simulink model "Simulateur_V8_eq06"  (R2024a)
settings: Solver=FixedStepAuto  StartTime=0.0  StopTime=1  FixedStep=1e-5  RelTol=1e-3
model workspace: external: MATLAB File Simulateur_V7_eq065_saveas.m (data not in the file)
values from neighbouring files (symbols this model uses):
  b = 72.82e-3    (= 0.07282)    [Init.m]    (also in Init_Complet.m)
  E = 18.6e9    (= 18600000000)    [Init.m]    (also in Init_Complet.m)
  h = 1.46e-3    (= 0.00146)    [Init.m]    (also in Init_Complet.m)
  L = 25e-2    (= 0.25)    [Init.m]    (also in Init_Complet.m)
  q = 0.14    [Init.m]    (also in Init_Complet.m)
undefined symbols (not defined in the file or in its folder): c, dens, m
libraries: simulink x3, slpidlib x2
settings Model: SimulationMode=accelerator  Creator=jeann  LastModifiedBy=dadah5
settings RTWCC: GPUComputeCapability=3.5

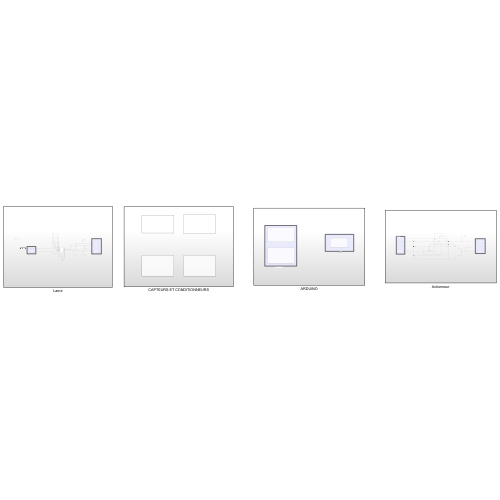
[thumbnail: Simulink's stored preview of the top-level diagram]
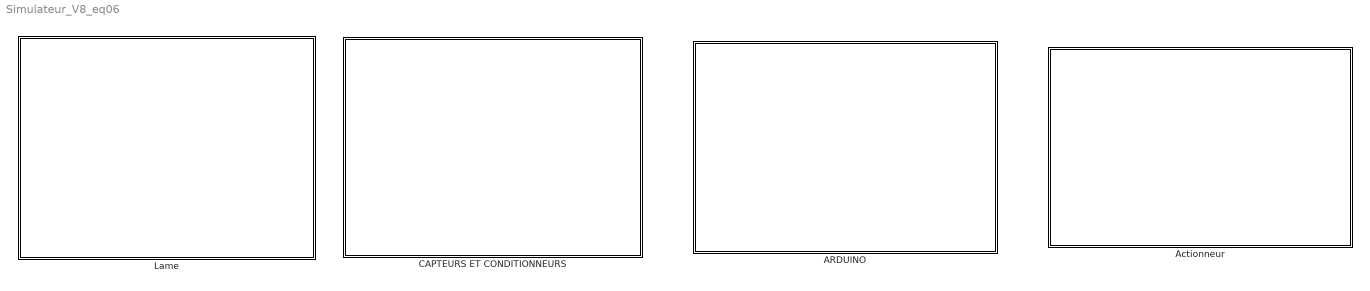
== system Simulateur_V8_eq06 ==
  ARDUINO : Subsystem
  Actionneur : Subsystem
  CAPTEURS ET CONDITIONNEURS : Subsystem
  Lame : Subsystem

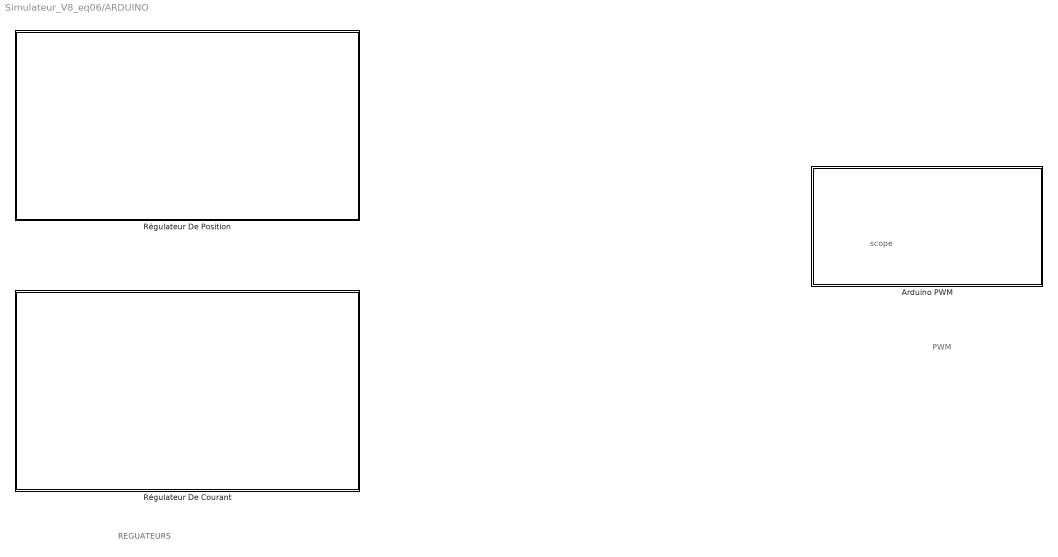
== system Simulateur_V8_eq06/ARDUINO ==
  note: scope
  note: REGUATEURS
  note: PWM
  Arduino PWM : Subsystem
  Régulateur De Courant : Subsystem
  Régulateur De Position : Subsystem

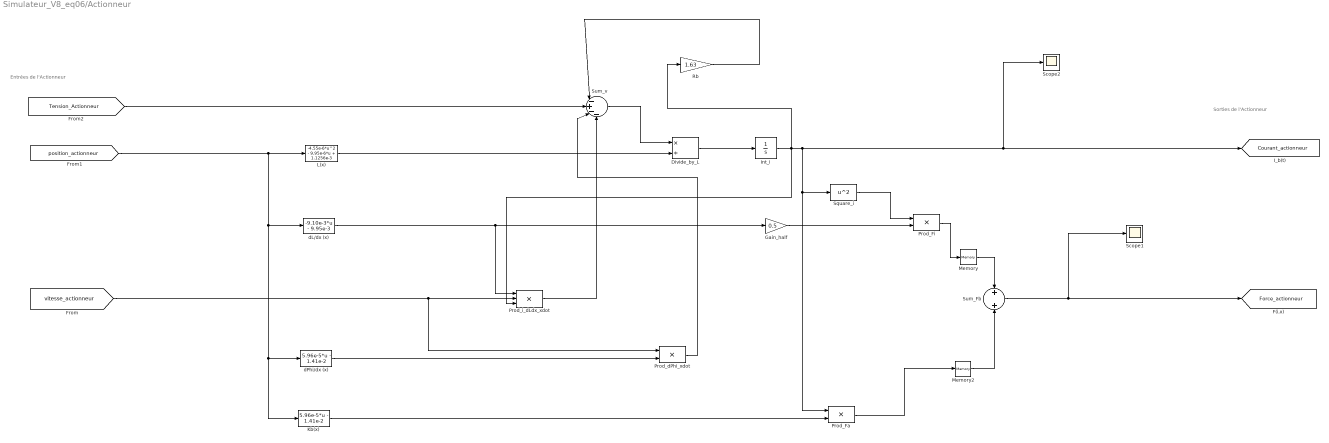
== system Simulateur_V8_eq06/Actionneur ==
  note: Sorties de l'Actionneur
  note: Entrées de l'Actionneur
  Divide_by_L : Product  Inputs=*/
  Gain_half : Gain  Gain=0.5
  Int_i : Integrator
  Kb(x) : Fcn  Expr=5.96e-5*u - 1.41e-2
  L(x) : Fcn  Expr=-4.55e-6*u^2 - 9.95e-6*u + 1.1256e-3
  Memory : Memory
  Memory2 : Memory
  Prod_Fa : Product
  Prod_Fi : Product
  Prod_dPhi_xdot : Product
  Prod_i_dLdx_xdot : Product  Inputs=3
  Rb : Gain  Gain=1.63
  Scope1 : Scope
  Scope2 : Scope
  Square_i : Math  Operator=square
  Sum_Fb : Sum
  Sum_v : Sum  Inputs=|-+--
  dL/dx (x) : Fcn  Expr=-9.10e-3*u - 9.95e-3
  dPhi/dx (x) : Fcn  Expr=5.96e-5*u - 1.41e-2
  tag scope: Courant_actionneur=global, Force_actionneur=global
  wires:
  dL/dx (x)/1 -> Gain_half/1, Prod_i_dLdx_xdot/1
  Sum_Fb/1 -> Scope1/1, [Force_actionneur]
  Rb/1 -> Sum_v/1
  Prod_i_dLdx_xdot/1 -> Sum_v/4
  L(x)/1 -> Divide_by_L/2
  Square_i/1 -> Prod_Fi/1
  Prod_dPhi_xdot/1 -> Sum_v/3
  Gain_half/1 -> Prod_Fi/2
  dPhi/dx (x)/1 -> Prod_dPhi_xdot/2
  Divide_by_L/1 -> Int_i/1
  Int_i/1 -> Prod_i_dLdx_xdot/3, Scope2/1, [Courant_actionneur], Square_i/1, Prod_Fa/1, Rb/1
  Sum_v/1 -> Divide_by_L/1
  [vitesse_actionneur] -> Prod_dPhi_xdot/1, Prod_i_dLdx_xdot/2
  Kb(x)/1 -> Prod_Fa/2
  [position_actionneur] -> dL/dx (x)/1, Kb(x)/1, dPhi/dx (x)/1, L(x)/1
  [Tension_Actionneur] -> Sum_v/2
  Prod_Fi/1 -> Memory/1
  Memory/1 -> Sum_Fb/1
  Prod_Fa/1 -> Memory2/1
  Memory2/1 -> Sum_Fb/2

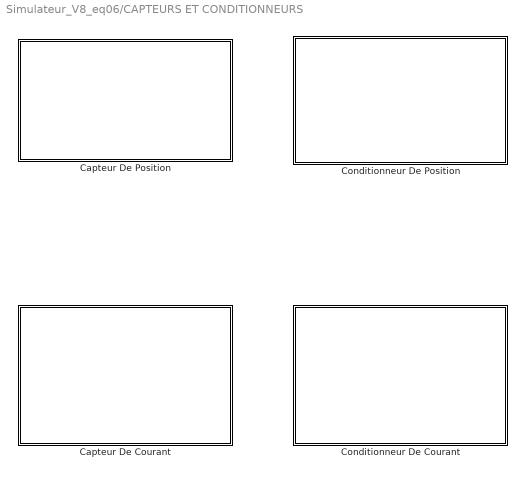
== system Simulateur_V8_eq06/CAPTEURS ET CONDITIONNEURS ==
  Capteur De Courant : Subsystem
  "Capteur De Position " : Subsystem
  Conditionneur De Courant : Subsystem
  Conditionneur De Position : Subsystem

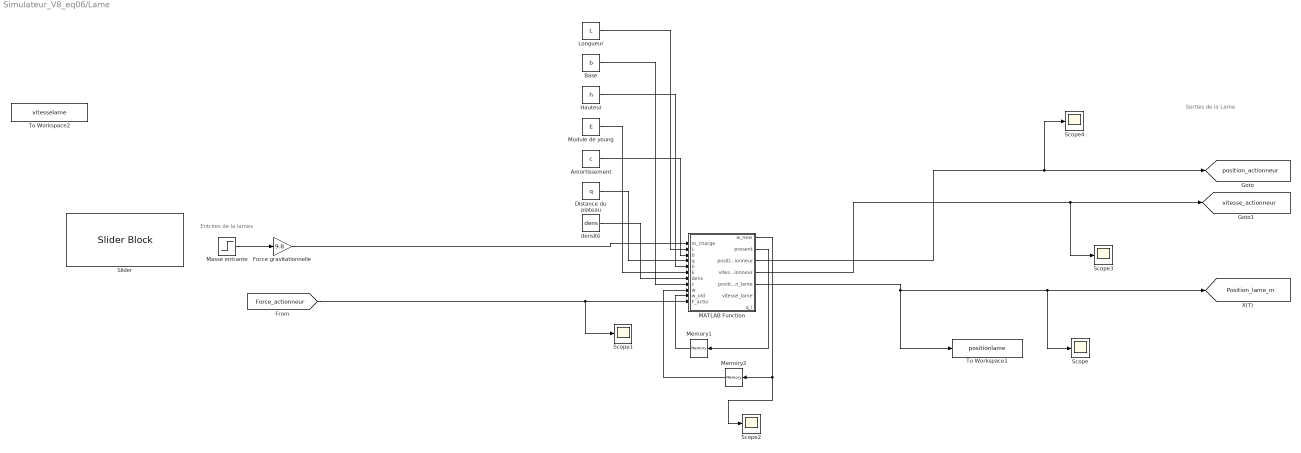
== system Simulateur_V8_eq06/Lame ==
  note: Sorties de la Lame
  note: Entrées de la lames
  Amortissement : Constant  Value=c
  Base : Constant  Value=b
  Distance du plateau : Constant  Value=q
  Force gravitationnelle : Gain  Gain=9.8
  Hauteur : Constant  Value=h
  Longueur : Constant  Value=L
  MATLAB Function : MATLAB Function  TreatAsAtomicUnit=on
  Masse entrante : Step  After=m  SampleTime=3
  Memory1 : Memory  InitialCondition=zeros(12,1)
  Memory2 : Memory  InitialCondition=zeros(12,1)  StateName=matrix
  Module de young : Constant  Value=E
  Scope{,1..4} (5 alike) : Scope
  Slider : SliderBlock
  To Workspace1 : ToWorkspace  VariableName=positionlame  SaveFormat=Timeseries  SampleTime=-1
  To Workspace2 : ToWorkspace  VariableName=vitesselame  SaveFormat=Timeseries  SampleTime=-1
  densité : Constant  Value=dens
  tag scope: Position_lame_m=global, position_actionneur=global, vitesse_actionneur=global
  wires:
  [Force_actionneur] -> Scope1/1, MATLAB Function/11(F_actio)
  MATLAB Function/1(w_new) -> Memory2/1, Scope2/1
  Memory2/1 -> MATLAB Function/9(w)
  MATLAB Function/2(present) -> Memory1/1
  Memory1/1 -> MATLAB Function/10(w_old)
  Hauteur/1 -> MATLAB Function/5(h)
  Module de young/1 -> MATLAB Function/6(E)
  Amortissement/1 -> MATLAB Function/3(b)
  Distance du plateau/1 -> MATLAB Function/4(q)
  densité/1 -> MATLAB Function/7(dens)
  Masse entrante/1 -> Force gravitationnelle/1
  Force gravitationnelle/1 -> MATLAB Function/1(m_charge)
  MATLAB Function/5(position_lame) -> To Workspace1/1, Scope/1, [Position_lame_m]
  MATLAB Function/4(vitesse_actionneur) -> Scope3/1, [vitesse_actionneur]
  MATLAB Function/3(position_actionneur) -> Scope4/1, [position_actionneur]
  Longueur/1 -> MATLAB Function/2(L)
  Base/1 -> MATLAB Function/8(c)

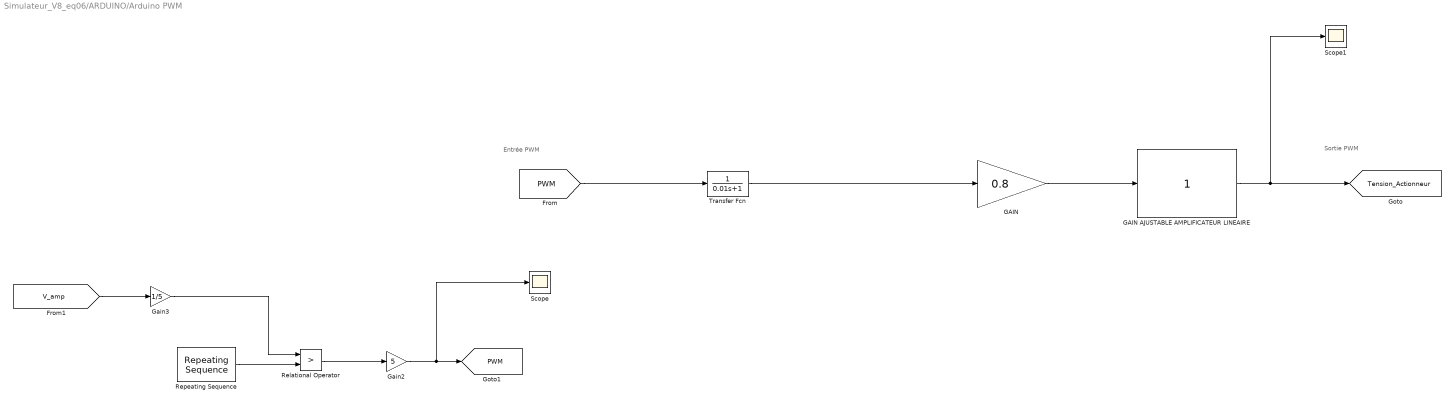
== system Simulateur_V8_eq06/ARDUINO/Arduino PWM ==
  note: Entrée PWM
  note: Sortie PWM
  GAIN : Gain  Gain=0.8
  GAIN AJUSTABLE AMPLIFICATEUR LINEAIRE : simulink/Math Operations/Slider Gain  gain=1  low=1  high=5
  Gain2 : Gain  Gain=5  ParamDataTypeStr=double
  Gain3 : Gain  Gain=1/5
  Relational Operator : RelationalOperator  Operator=>  OutDataTypeStr=boolean  RndMeth=Simplest  InputSameDT=off
  Repeating Sequence : simulink/Sources/Repeating Sequence  rep_seq_t=[0 0.001 0.002]  rep_seq_y=[0 1 0]
  Scope : Scope
  Scope1 : Scope
  Transfer Fcn : TransferFcn  Denominator=[0.01 1]
  tag scope: PWM=global, Tension_Actionneur=global
  wires:
  Transfer Fcn/1 -> GAIN/1
  GAIN AJUSTABLE AMPLIFICATEUR LINEAIRE/1 -> Scope1/1, [Tension_Actionneur]
  GAIN/1 -> GAIN AJUSTABLE AMPLIFICATEUR LINEAIRE/1
  Repeating Sequence/1 -> Relational Operator/2
  Relational Operator/1 -> Gain2/1
  Gain2/1 -> Scope/1, [PWM]
  [PWM] -> Transfer Fcn/1
  [V_amp] -> Gain3/1
  Gain3/1 -> Relational Operator/1

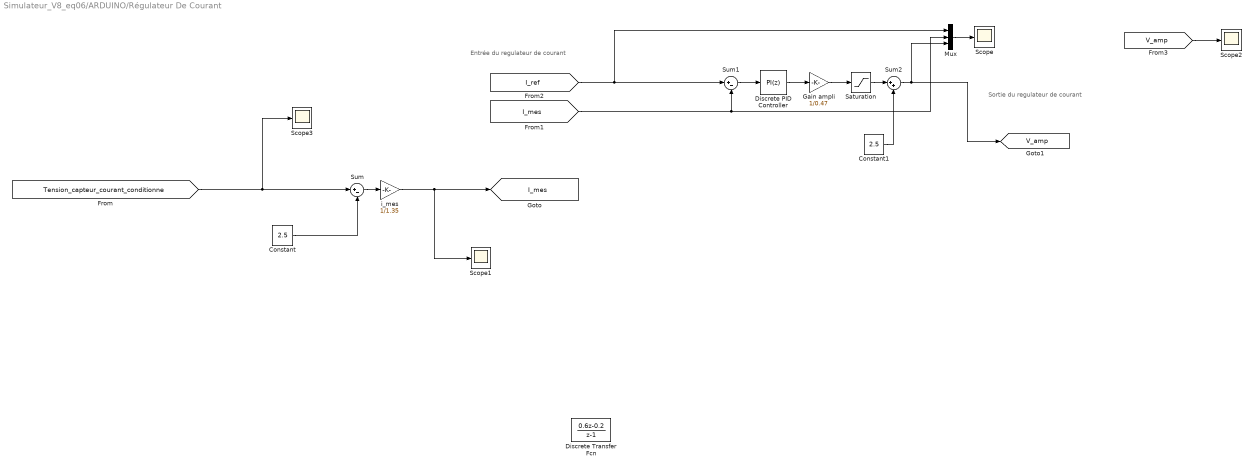
== system Simulateur_V8_eq06/ARDUINO/Régulateur De Courant ==
  note: Entrée du regulateur de courant
  note: Sortie du regulateur de courant
  Constant : Constant  Value=2.5
  Constant1 : Constant  Value=2.5
  Discrete Transfer Fcn : DiscreteTransferFcn  Numerator="[0.6  -0.2]"  Denominator="[1  -1]"
  Discrete PID Controller : slpidlib/PID Controller  Controller=PI  Form=Parallel  TimeDomain=Discrete-time  UseExternalTs=off  SampleTime=0.002  IntegratorMethod=Forward Euler  FilterMethod=Forward Euler  ControllerParametersSource=internal  P=0.18  I=180  UseKiTs=off  D=0  UseExternalDerivativeSource=off  N=100  UseFilter=on  TunerSelectOption=Transfer Function Based (PID Tuner App)  InitialConditionSource=internal  InitialConditionForIntegrator=0  InitialConditionForFilter=0  DifferentiatorICPrevScaledInput=0  ExternalReset=none  TrackingMode=off  Kt=1  LimitOutput=on  SatLimitsSource=internal  UpperSaturationLimit=5  LowerSaturationLimit=-5  LinearizeAsGain=off  AntiWindupMode=back-calculation  Kb=1  LimitIntegrator=off  UpperIntegratorSaturationLimit=inf  LowerIntegratorSaturationLimit=-inf  POutMin=[]  POutMax=[]  IOutMin=[]  IOutMax=[]  DOutMin=[]  DOutMax=[]  NOutMin=[]  NOutMax=[]  SumOutMin=[]  SumOutMax=[]  SaturationOutMin=[]  SaturationOutMax=[]  PParamMin=[]  PParamMax=[]  IParamMin=[]  IParamMax=[]  DParamMin=[]  DParamMax=[]  NParamMin=[]  NParamMax=[]  KbParamMin=[]  KbParamMax=[]  KtParamMin=[]  KtParamMax=[]  KbOutMin=[]  KbOutMax=[]  KtOutMin=[]  KtOutMax=[]  IntegratorOutMin=[]  IntegratorOutMax=[]  FilterOutMin=[]  FilterOutMax=[]  SumI1OutMin=[]  SumI1OutMax=[]  SumI2OutMin=[]  SumI2OutMax=[]  SumI3OutMin=[]  SumI3OutMax=[]  SumI4OutMin=[]  SumI4OutMax=[]  SumDOutMin=[]  SumDOutMax=[]  DifferentiatorOutMin=[]  DifferentiatorOutMax=[]  FilterDiffOutCoefMin=[]  FilterDiffOutCoefMax=[]  ReciprocalOutMin=[]  ReciprocalOutMax=[]  SumDenOutMin=[]  SumDenOutMax=[]  SumNumOutMin=[]  SumNumOutMax=[]  DivideOutMin=[]  DivideOutMax=[]  UdiffTsProdOutMin=[]  UdiffTsProdOutMax=[]  NTsProdOutMin=[]  NTsProdOutMax=[]  UintegralTsProdOutMin=[]  UintegralTsProdOutMax=[]  UngainTsProdOutMin=[]  UngainTsProdOutMax=[]  ClampingZeroOutDataTypeStr=Inherit: Inherit via back propagation  ClampingZeroOutMin=[]  ClampingZeroOutMax=[]  FilterDenConstantOutDataTypeStr=Inherit: Inherit via back propagation  FilterDenConstantOutMin=[]  FilterDenConstantOutMax=[]  PCopyOutDataTypeStr=Inherit: Inherit via back propagation  PCopyOutMin=[]  PCopyOutMax=[]  NCopyOutDataTypeStr=Inherit: Inherit via back propagation  NCopyOutMin=[]  NCopyOutMax=[]  IntegratorContinuousStateAttributes=''  IntegratorStateMustResolveToSignalObject=off  IntegratorRTWStateStorageClass=Auto  FilterContinuousStateAttributes=''  FilterStateMustResolveToSignalObject=off  FilterRTWStateStorageClass=Auto  ParallelPVariant=InternalParameters  IdealPVariant=Disabled  IVariant=InternalParameters  DVariant=Disabled  IntegratorVariant=Discrete  SatVariant=Enabled  AWVariant=BackCalculation  PCopyVariant=Disabled  TRVariant=Disabled  FdbkBlocksVariant=Forward  IdealPFdbkVariant=Disabled  SatFdbkVariant=Disabled  DerivativeFilterVariant=Disabled  NVariant=Disabled  NCopyVariant=Disabled_SignalSpec  FilterICVariant=Disabled  IntegratorICVariant=InternalICs  ExternalResetVariant=Disabled  TRSumVariant=Passthrough  SumFdbkVariant=Disabled  SumVariant=Sum_PI  TsampFilterVariant=InternalTs  TsampNgainVariant=Passthrough  TsampIntegralVariant=Disabled_SignalSpec  ExternalSaturationOutDataTypeStr=Inherit: Same as second input  DerivativeSourceVariant=Disabled
      settings: LibrarySourceBlock=simulink/Discrete/Discrete PID Controller
  "Gain ampli " : Gain  Gain=1/0.47
  Mux : Mux  Inputs=3
  Saturation : Saturate  UpperLimit=5  LowerLimit=0
  Scope{,1..3} (4 alike) : Scope
  Sum : Sum  Inputs=|+-
  Sum1 : Sum  Inputs=|+-
  Sum2 : Sum  Inputs=|++
  i_mes : Gain  Gain=1/1.35
  tag scope: I_mes=global, V_amp=global
  wires:
  [I_ref] -> Mux/1, Sum1/1
  Saturation/1 -> Sum2/1
  Constant1/1 -> Sum2/2
  Constant/1 -> Sum/2
  [Tension_capteur_courant_conditionne] -> Scope3/1, Sum/1
  Sum/1 -> i_mes/1
  Mux/1 -> Scope/1
  Sum2/1 -> [V_amp], Mux/3
  i_mes/1 -> Scope1/1, [I_mes]
  [I_mes] -> Sum1/2, Mux/2
  Sum1/1 -> Discrete PID Controller/1
  Discrete PID Controller/1 -> "Gain ampli "/1
  [V_amp] -> Scope2/1
  "Gain ampli "/1 -> Saturation/1

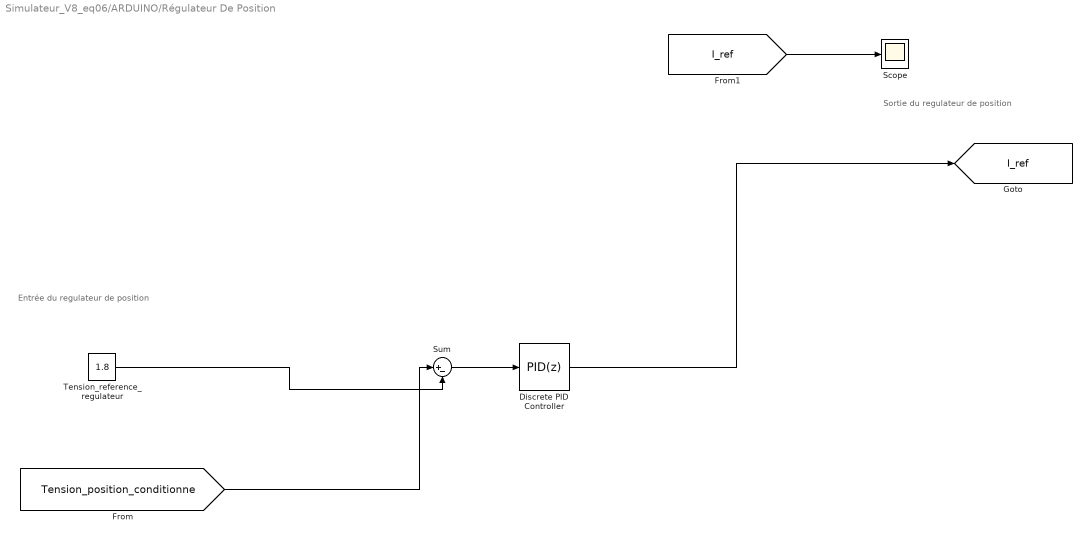
== system Simulateur_V8_eq06/ARDUINO/Régulateur De Position ==
  note: Entrée du regulateur de position
  note: Sortie du regulateur de position
  Discrete PID Controller : slpidlib/PID Controller  Controller=PID  Form=Parallel  TimeDomain=Discrete-time  UseExternalTs=off  SampleTime=0.002  IntegratorMethod=Forward Euler  FilterMethod=Forward Euler  ControllerParametersSource=internal  P=0.85  I=2.8333  UseKiTs=off  D=0.017  UseExternalDerivativeSource=off  N=100  UseFilter=on  TunerSelectOption=Transfer Function Based (PID Tuner App)  InitialConditionSource=internal  InitialConditionForIntegrator=0  InitialConditionForFilter=0  DifferentiatorICPrevScaledInput=0  ExternalReset=none  TrackingMode=off  Kt=1  LimitOutput=on  SatLimitsSource=internal  UpperSaturationLimit=2.9  LowerSaturationLimit=-2.9  LinearizeAsGain=off  AntiWindupMode=back-calculation  Kb=1  LimitIntegrator=off  UpperIntegratorSaturationLimit=inf  LowerIntegratorSaturationLimit=-inf  POutMin=[]  POutMax=[]  IOutMin=[]  IOutMax=[]  DOutMin=[]  DOutMax=[]  NOutMin=[]  NOutMax=[]  SumOutMin=[]  SumOutMax=[]  SaturationOutMin=[]  SaturationOutMax=[]  PParamMin=[]  PParamMax=[]  IParamMin=[]  IParamMax=[]  DParamMin=[]  DParamMax=[]  NParamMin=[]  NParamMax=[]  KbParamMin=[]  KbParamMax=[]  KtParamMin=[]  KtParamMax=[]  KbOutMin=[]  KbOutMax=[]  KtOutMin=[]  KtOutMax=[]  IntegratorOutMin=[]  IntegratorOutMax=[]  FilterOutMin=[]  FilterOutMax=[]  SumI1OutMin=[]  SumI1OutMax=[]  SumI2OutMin=[]  SumI2OutMax=[]  SumI3OutMin=[]  SumI3OutMax=[]  SumI4OutMin=[]  SumI4OutMax=[]  SumDOutMin=[]  SumDOutMax=[]  DifferentiatorOutMin=[]  DifferentiatorOutMax=[]  FilterDiffOutCoefMin=[]  FilterDiffOutCoefMax=[]  ReciprocalOutMin=[]  ReciprocalOutMax=[]  SumDenOutMin=[]  SumDenOutMax=[]  SumNumOutMin=[]  SumNumOutMax=[]  DivideOutMin=[]  DivideOutMax=[]  UdiffTsProdOutMin=[]  UdiffTsProdOutMax=[]  NTsProdOutMin=[]  NTsProdOutMax=[]  UintegralTsProdOutMin=[]  UintegralTsProdOutMax=[]  UngainTsProdOutMin=[]  UngainTsProdOutMax=[]  ClampingZeroOutDataTypeStr=Inherit: Inherit via back propagation  ClampingZeroOutMin=[]  ClampingZeroOutMax=[]  FilterDenConstantOutDataTypeStr=Inherit: Inherit via back propagation  FilterDenConstantOutMin=[]  FilterDenConstantOutMax=[]  PCopyOutDataTypeStr=Inherit: Inherit via back propagation  PCopyOutMin=[]  PCopyOutMax=[]  NCopyOutDataTypeStr=Inherit: Inherit via back propagation  NCopyOutMin=[]  NCopyOutMax=[]  IntegratorContinuousStateAttributes=''  IntegratorStateMustResolveToSignalObject=off  IntegratorRTWStateStorageClass=Auto  FilterContinuousStateAttributes=''  FilterStateMustResolveToSignalObject=off  FilterRTWStateStorageClass=Auto  ParallelPVariant=InternalParameters  IdealPVariant=Disabled  IVariant=InternalParameters  DVariant=InternalParameters  IntegratorVariant=Discrete  SatVariant=Enabled  AWVariant=BackCalculation  PCopyVariant=Disabled  TRVariant=Disabled  FdbkBlocksVariant=Forward  IdealPFdbkVariant=Disabled  SatFdbkVariant=Disabled  DerivativeFilterVariant=ForwardEulerFilter  NVariant=InternalParameters  NCopyVariant=Disabled  FilterICVariant=InternalICsFilter  IntegratorICVariant=InternalICs  ExternalResetVariant=Disabled  TRSumVariant=Passthrough  SumFdbkVariant=Disabled  SumVariant=Sum_PID  TsampFilterVariant=InternalTs  TsampNgainVariant=Passthrough  TsampIntegralVariant=Disabled_SignalSpec  ExternalSaturationOutDataTypeStr=Inherit: Same as second input  DerivativeSourceVariant=ErrorSignal
      settings: LibrarySourceBlock=simulink/Discrete/Discrete PID Controller
  Scope : Scope
  Sum : Sum  Inputs=|+-
  Tension_reference_regulateur : Constant  Value=1.8
  tag scope: I_ref=global
  wires:
  Sum/1 -> Discrete PID Controller/1
  Tension_reference_regulateur/1 -> Sum/2
  [Tension_position_conditionne] -> Sum/1
  Discrete PID Controller/1 -> [I_ref]
  [I_ref] -> Scope/1

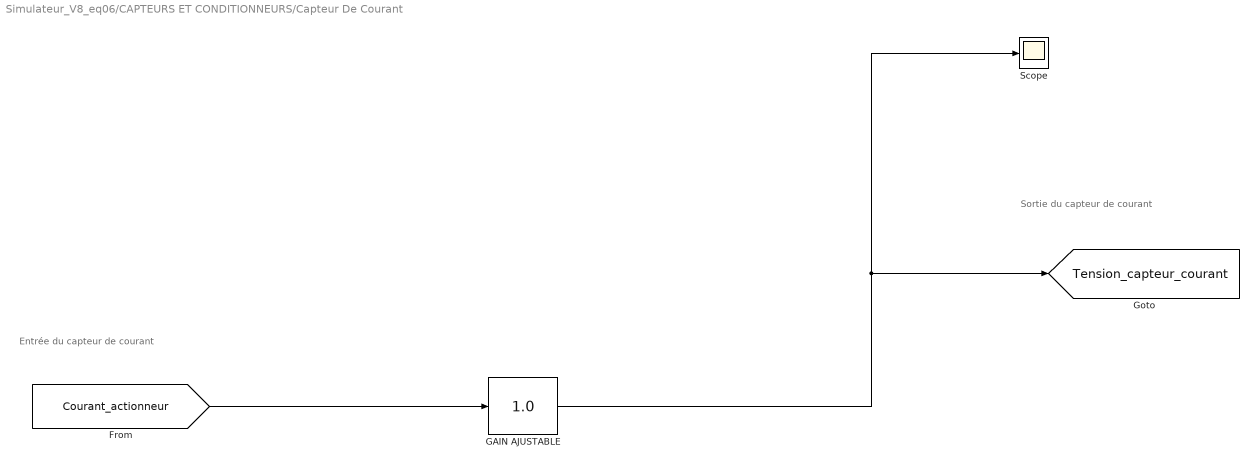
== system Simulateur_V8_eq06/CAPTEURS ET CONDITIONNEURS/Capteur De Courant ==
  note: Sortie du capteur de courant
  note: Entrée du capteur de courant
  GAIN AJUSTABLE : simulink/Math Operations/Slider Gain  gain=1.0  low=1  high=10
  Scope : Scope
  tag scope: Tension_capteur_courant=global
  wires:
  [Courant_actionneur] -> GAIN AJUSTABLE/1
  GAIN AJUSTABLE/1 -> Scope/1, [Tension_capteur_courant]

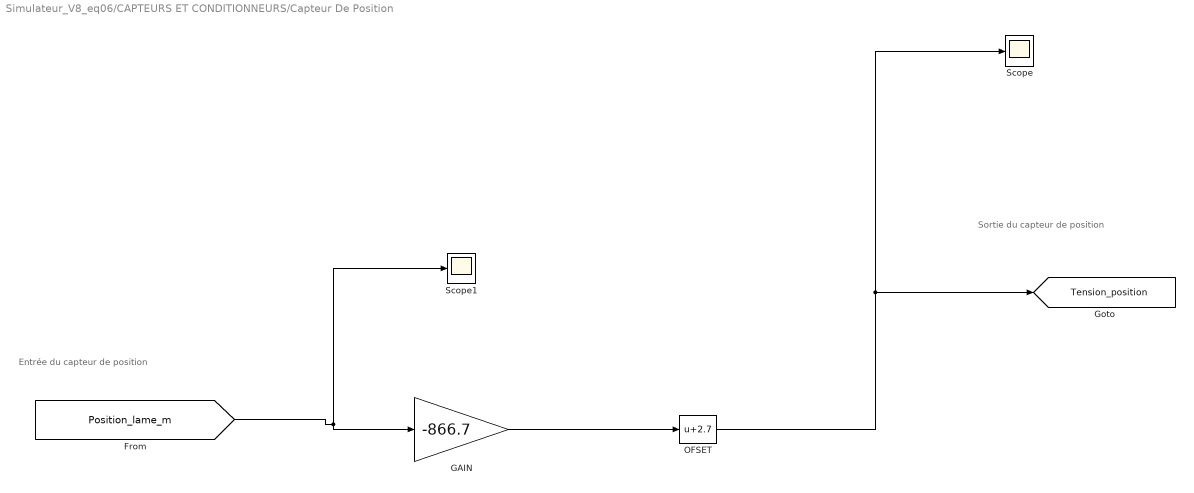
== system Simulateur_V8_eq06/CAPTEURS ET CONDITIONNEURS/Capteur De Position  ==
  note: Entrée du capteur de position
  note: Sortie du capteur de position
  GAIN : Gain  Gain=-866.7
  OFSET : Bias  Bias=2.7  SaturateOnIntegerOverflow=off
  Scope : Scope
  Scope1 : Scope
  tag scope: Tension_position=global
  wires:
  [Position_lame_m] -> GAIN/1, Scope1/1
  GAIN/1 -> OFSET/1
  OFSET/1 -> Scope/1, [Tension_position]

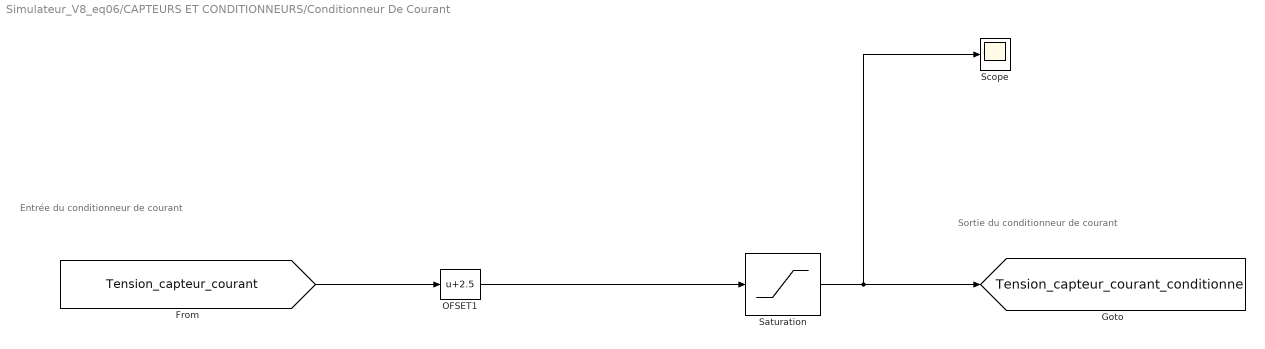
== system Simulateur_V8_eq06/CAPTEURS ET CONDITIONNEURS/Conditionneur De Courant ==
  note: Sortie du conditionneur de courant
  note: Entrée du conditionneur de courant
  OFSET1 : Bias  Bias=2.5  SaturateOnIntegerOverflow=off
  Saturation : Saturate  UpperLimit=4.5  LowerLimit=0.5
  Scope : Scope
  tag scope: Tension_capteur_courant_conditionne=global
  wires:
  [Tension_capteur_courant] -> OFSET1/1
  Saturation/1 -> Scope/1, [Tension_capteur_courant_conditionne]
  OFSET1/1 -> Saturation/1

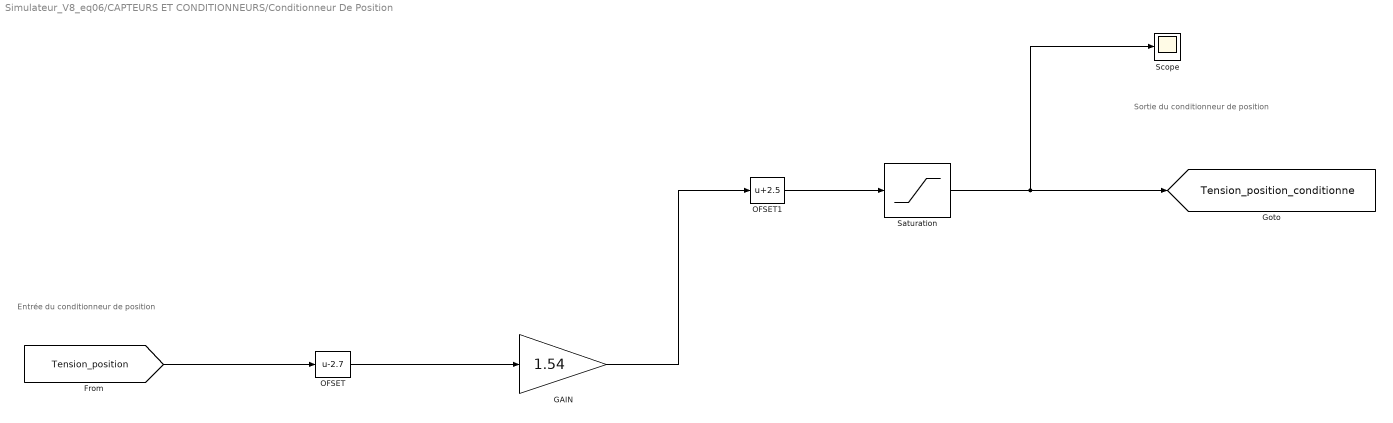
== system Simulateur_V8_eq06/CAPTEURS ET CONDITIONNEURS/Conditionneur De Position ==
  note: Sortie du conditionneur de position
  note: Entrée du conditionneur de position
  GAIN : Gain  Gain=1.54
  OFSET : Bias  Bias=-2.7  SaturateOnIntegerOverflow=off
  OFSET1 : Bias  Bias=2.5  SaturateOnIntegerOverflow=off
  Saturation : Saturate  UpperLimit=5  LowerLimit=0
  Scope : Scope
  tag scope: Tension_position_conditionne=global
  wires:
  OFSET/1 -> GAIN/1
  GAIN/1 -> OFSET1/1
  OFSET1/1 -> Saturation/1
  Saturation/1 -> Scope/1, [Tension_position_conditionne]
  [Tension_position] -> OFSET/1

== matlab function Simulateur_V8_eq06/Lame/MATLAB Function ==
  data: m_charge input; L input; b input; q input; h input; E input; dens input; c input; w_new output; w input; w_old input; present output; position_actionneur output; vitesse_actionneur output; position_lame output; vitesse_lame output; F_actio input; q_i output
function [w_new, present, position_actionneur, vitesse_actionneur, position_lame, vitesse_lame, q_i] = fcn(m_charge, L, b, q, h, E, dens, c, w, w_old, F_actio)

% =========================
% Paramètres de la poutre
% =========================
J = b*h^3/12;          % Moment quadratique de la section [m^4]
mu = dens*b*h;         % Masse linéique [kg/m]

% =========================
% Paramètres physiques
% =========================
m_lame   = mu*L;       % Masse totale approximative de la lame [kg]
m_aimant = 9.3e-3;     % Masse de l'aimant [kg]
g = -9.8;              % Gravité [m/s^2]
dt = 1e-5;             % Pas de temps [s]

% =========================
% Discrétisation spatiale
% =========================
nx = 10;               % Nombre de noeuds internes utiles
dx = L/(nx-1);         % Pas spatial [m]

% Position discrète de la masse / force appliquée
q_i = 2 + round(q/dx);

% Ajout de 2 noeuds fantômes pour les conditions limites
nx = nx + 2;

% Sécurité pour éviter de sortir des bornes utiles
q_i = max(3, min(q_i, nx-2));

% =========================
% Mise en forme des états
% =========================
w     = w(:);
w_old = w_old(:);

if length(w) ~= nx
    w = zeros(nx,1);
end

if length(w_old) ~= nx
    w_old = zeros(nx,1);
end

% =========================
% Vecteur des forces
% =========================
F = zeros(nx,1);
F(end) = g*m_aimant;                 % Poids de l'aimant au bout
F(q_i) = g*m_charge + F_actio;       % Poids de la charge + force actionneur

% =========================
% Coefficients de calcul
% =========================
coeff1   = -E*J*dt^2/(mu*dx^4); % Coefficient de rigidité (flexion de la poutre) : traduit l'effet du terme EI*d^4w/dx^4 sur la déformation
coeff_amt = c*dt/mu;            % Coefficient d’amortissement : modélise les pertes d’énergie (proportionnel à la vitesse (w - w_old))
coeff_F  = dt^2/(mu*dx);        % Coefficient de force : transforme la force appliquée F(i) en déplacement de la lame

% =========================
% Initialisation
% =========================
w_new = zeros(nx,1);

% =========================
% Mise à jour de la déformation
% =========================
i = 3:nx-2;

w_new(i) = ...
    coeff1 * ( w(i+2) - 4*w(i+1) + 6*w(i) - 4*w(i-1) + w(i-2) ) ...
    + 2*w(i) - w_old(i) ...
    - coeff_amt * (w(i) - w_old(i)) ...
    + coeff_F * F(i);

% =========================
% Conditions limites
% =========================
w_new(1:2) = 0;    % Encastrement : déplacement et pente nuls

% Extrémité libre : dérivées 2e et 3e nulles
w_new(end-1) = 2*w_new(end-2) - w_new(end-3);
w_new(end)   = 2*w_new(end-1) - w_new(end-2);

% =========================
% Sorties
% =========================
present = w;                                      % Etat actuel pour mémoire

% Sorties pour l'actionneur (au noeud q_i)
position_actionneur = w_new(q_i);                 
vitesse_actionneur  = (w_new(q_i) - w(q_i))/dt;  

% Sorties pour le capteur de position (au bout de la lame)
position_lame = w_new(end);                       
vitesse_lame  = (w_new(end) - w(end))/dt;         

end
